simulink model "UKF_slopeestimation"  (R2019b)
settings: Solver=VariableStepAuto  StartTime=0.0  StopTime=4.0  FixedStep=0.05  RelTol=1e-3
settings Model: Creator=win10  LastModifiedBy=win10

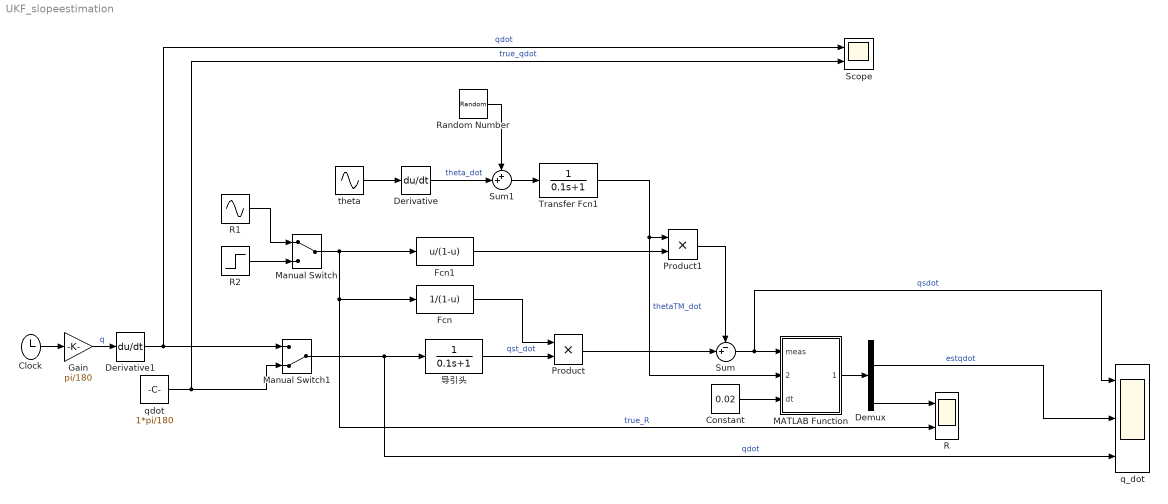
== system UKF_slopeestimation ==
  Clock : Clock
  Constant : Constant  Value=0.02
  Demux : Demux
  Derivative : Derivative
  Derivative1 : Derivative
  Fcn : Fcn  Expr=1/(1-u)
  Fcn1 : Fcn  Expr=u/(1-u)
  Gain : Gain  Gain=pi/180
  MATLAB Function : MATLAB Function  TreatAsAtomicUnit=on
  Manual Switch : ManualSwitch
  Manual Switch1 : ManualSwitch  CurrentSetting=0
  Product : Product
  Product1 : Product
  R : Scope  NumInputPorts=2
  R1 : Sin  Amplitude=0.06  Frequency=pi  SampleTime=0
  R2 : Step  Time=2  Before=0.06  After=0.03  SampleTime=0
  Random Number : RandomNumber  Variance=0.04*pi*pi/180/180  SampleTime=0.1
  Scope : Scope  NumInputPorts=2
  Sum : Sum  Inputs=-+|
  Sum1 : Sum  Inputs=++|
  Transfer Fcn1 : TransferFcn  Denominator=[0.1 1]
  q_dot : Scope  NumInputPorts=3
  qdot : Constant  Value=1*pi/180
  theta : Sin  Amplitude=3*pi/180  Frequency=4*pi  SampleTime=0
  导引头 : TransferFcn  Denominator=[0.1 1]
  wires:
  导引头/1 -> Product/2  "qst_dot"
  Fcn/1 -> Product/1
  Product/1 -> Sum/2
  Sum1/1 -> Transfer Fcn1/1
  Random Number/1 -> Sum1/1
  Fcn1/1 -> Product1/2
  Transfer Fcn1/1 -> MATLAB Function/2(thetaTM_dot), Product1/1  "thetaTM_dot"
  Product1/1 -> Sum/1
  Derivative/1 -> Sum1/2  "theta_dot"
  theta/1 -> Derivative/1
  Sum/1 -> q_dot/1, MATLAB Function/1(meas)  "qsdot"
  MATLAB Function/1(xhatOut) -> Demux/1
  Demux/4 -> R/1
  R2/1 -> Manual Switch/2
  R1/1 -> Manual Switch/1
  Manual Switch/1 -> R/2, Fcn/1, Fcn1/1  "true_R"
  Derivative1/1 -> Manual Switch1/1, Scope/1  "qdot"
  qdot/1 -> Manual Switch1/2, Scope/2  "true_qdot"
  Gain/1 -> Derivative1/1  "q"
  Clock/1 -> Gain/1
  Constant/1 -> MATLAB Function/3(dt)
  Manual Switch1/1 -> q_dot/3, 导引头/1  "qdot"
  Demux/2 -> q_dot/2  "estqdot"

== matlab function UKF_slopeestimation/MATLAB Function ==
  settings: updateMethod=DISCRETE  sampleTime=0.02
  data: meas input; xhatOut output; thetaTM_dot input; dt input
function xhatOut = UKF_Simulink(meas,thetaTM_dot,dt)
% This Embedded MATLAB Function implements an unscented Kalman filter used
% for target tracking.
%
% The continuous-time process model is given by
% dx/dt = f(x(t)) + w(t)

% where, x(t) = [q q_dot qst_dot rou]', q,q_dot is true LOS angle and LOS rate 
% qst_dot is true output of LOS rate from seeker, rou is the radome error
% slope. w(t) = [0 w2(t) 0  w4(t)]'


% and the measurements are given by
% y = qst_dot/(1-rou) - rou/(1-rou)*thetaTM_dot

% Define storage for the variables that need to persist
% between time periods.
Td = 0.1;

%% initialization

persistent P xhat Q R
if isempty(P)
 xhat = [0;0;0;0];
 P = diag([1 1 1 0.0005]);
 Q = diag([0 1e-5 0 1e-3]);
 R = diag([0.04*pi*pi/180/180]);
end

%% start UKF

n = numel(xhat);                                 %number of states
m = numel(meas);                                 %number of measurements
alpha = 1e-3;                                    %default, tunable
ki = 0;                                          %default, tunable
beta = 2;                                        %default, tunable
lambda = alpha^2*(n+ki)-n;                       %scaling factor
c = n+lambda;                                    %scaling factor
sigma = zeros(n,2*n);
sigma_prior = zeros(n,2*n);

% sigma points of previous state
Wm = [lambda/c 0.5/c+zeros(1,2*n)];              %weights for means 1*(1+2*n)******
Wc = Wm;
Wc(1) = Wc(1)+(1-alpha^2+beta);                  %weights for covariance
[root,~] = chol(c*P);
 for i = 1 : n
       sigma(:,i) = xhat + root(i,:)';
       sigma(:,i+n) = xhat - root(i,:)';
 end
xsigma = [xhat sigma];

% UKF time update
L = size(xsigma,2); 
xprior = zeros(n,1);
for i = 1 : L
    for tau = dt/10 : dt/10 : dt
        xsigma(1,i) = xsigma(1,i) + xsigma(2,i) * dt/10;
        xsigma(2,i) = xsigma(2,i) + 0 * dt/10;
        xsigma(3,i) = xsigma(3,i) + (xsigma(2,i)/Td - xsigma(3,i)/Td) * dt/10;
        xsigma(4,i) = xsigma(4,i) + 0 * dt/10;
    end
    xprior = xprior + Wm(i) * xsigma(:,i);
end
Pprior = zeros(n,n);
for i = 1 : L
    Pprior = Pprior + Wc(i) * (xsigma(:,i) - xprior) * (xsigma(:,i) - xprior)';
end
Pprior = Pprior + Q;

% UKF measurement update
% sigma points of prior state, can be omitted
[root_prior,~] = chol(c*Pprior);
 for i = 1 : n
       sigma_prior(:,i) = xprior + root_prior(i,:)';
       sigma_prior(:,i+n) = xprior - root_prior(i,:)';
 end
xsigma = [xprior sigma_prior];
% measurement prediction
yhat = zeros(m,1);
ysigma = zeros(m,L);
for i = 1 : L
      ysigma(:,i) = xsigma(3,i)/(1-xsigma(4,i)) - xsigma(4,i)/(1-xsigma(4,i))*thetaTM_dot;
      yhat = yhat + Wm(i) * ysigma(:,i);
end
 Pyy = zeros(m,m);
 Pxy = zeros(n,m);
 for i = 1 : L
      Pyy = Pyy + Wc(i) * (ysigma(:,i) - yhat) *  (ysigma(:,i) - yhat)';
      Pxy = Pxy + Wc(i) * (xsigma(:,i) - xprior) *  (ysigma(:,i) - yhat)';%****
  end  
  Pyy = Pyy + R;
  % filter gain
  Kukf = Pxy * inv(Pyy);
  xhat = xprior + Kukf * (meas - yhat);
  P = Pprior - Kukf * Pyy * Kukf';   
  
% Post the results
xhatOut = xhat;
